simulink model "carModelMPC"  (R2020a)
settings: Solver=FixedStepAuto  StartTime=0.0  StopTime=time_length1  FixedStep=0.01  RelTol=1e-3
values from neighbouring files (symbols this model uses):
  c_s = 1450    [main_file.m]
  k_s = 30.01e+3    (= 30010)    [main_file.m]
  k_t = 3.4e5    (= 340000)    [main_file.m]
  m_s = 395.3    [main_file.m]
  m_u = 48.3    [main_file.m]
  P_dis = c2d(P,ts)    [main_file.m]
  ts = 0.01    [main_file.m]
undefined symbols (not defined in the file or in its folder): F_lim
settings Model: Creator=20183992  LastModifiedBy=Harold
settings DataIOCC: SaveFormat=Array  ReturnWorkspaceOutputs=off
settings DebuggingCC: ArithmeticOperatorsInVariantConditions=warning
settings SFSimCC: SimUseLocalCustomCode=off  CustomCodeUndefinedFunction=UseInterfaceOnly
settings RTWCC: RTWUseLocalCustomCode=off

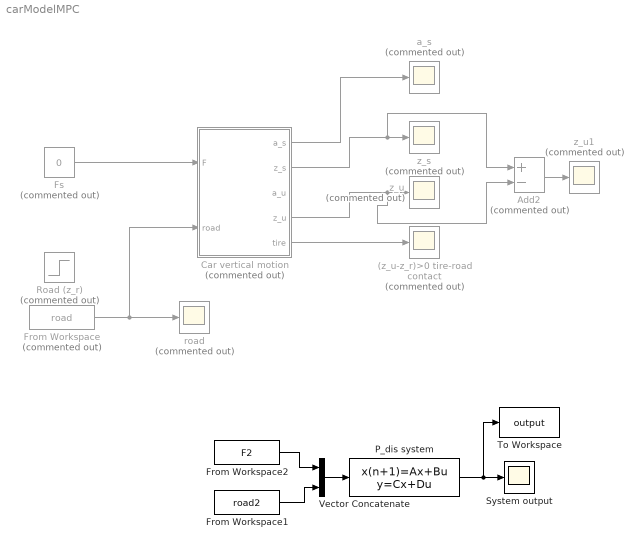
== system carModelMPC ==
  (z_u-z_r)>0 tire-road contact : Scope  Commented=on
  Add2 : Sum  Commented=on  Inputs=+-
  Car vertical motion : Subsystem  Commented=on
  From Workspace : FromWorkspace  Commented=on  VariableName=road  OutDataTypeStr=double  SampleTime=-1
  From Workspace1 : FromWorkspace  VariableName=road2  OutDataTypeStr=double  SampleTime=0.01
  From Workspace2 : FromWorkspace  VariableName=F2  OutDataTypeStr=double  SampleTime=0.01
  Fs : Constant  Commented=on  Value=0
  P_dis system : DiscreteStateSpace  A=P_dis.A  B=P_dis.B  C=P_dis.C  D=P_dis.D  SampleTime=ts
  Road (z_r) : Step  Commented=on  After=-0.1  SampleTime=0
  System output : Scope
  To Workspace : ToWorkspace  VariableName=output  SaveFormat=Timeseries  SampleTime=0.01
  Vector Concatenate : Concatenate  ConcatenateDimension=2
  a_s : Scope  Commented=on
  road : Scope  Commented=on
  z_s : Scope  Commented=on
  z_u : Scope  Commented=on
  z_u1 : Scope  Commented=on
  wires:
  Fs/1 -> Car vertical motion/1(F)
  Car vertical motion/5(tire) -> (z_u-z_r)>0 tire-road contact/1
  Car vertical motion/2(z_s) -> Add2/1, z_s/1
  Car vertical motion/4(z_u) -> Add2/2, z_u/1
  From Workspace/1 -> Car vertical motion/2(road), road/1
  Car vertical motion/1(a_s) -> a_s/1
  Add2/1 -> z_u1/1
  P_dis system/1 -> To Workspace/1, System output/1
  Vector Concatenate/1 -> P_dis system/1
  From Workspace1/1 -> Vector Concatenate/2
  From Workspace2/1 -> Vector Concatenate/1

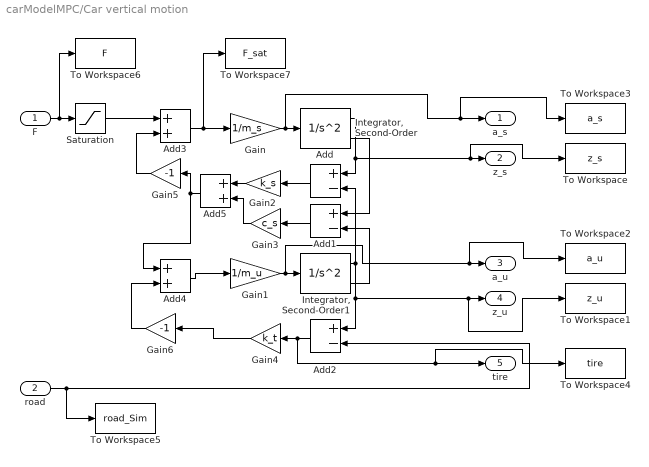
== system carModelMPC/Car vertical motion ==
  F : Inport
  road : Inport  Port=2
  Add : Sum  Inputs=+-
  Add1 : Sum  Inputs=+-
  Add2 : Sum  Inputs=+-
  Add3 : Sum
  Add4 : Sum
  Add5 : Sum
  Gain : Gain  Gain=1/m_s
  Gain1 : Gain  Gain=1/m_u
  Gain2 : Gain  Gain=k_s
  Gain3 : Gain  Gain=c_s
  Gain4 : Gain  Gain=k_t
  Gain5 : Gain  Gain=-1
  Gain6 : Gain  Gain=-1
  "Integrator, Second-Order" : SecondOrderIntegrator
  "Integrator, Second-Order1" : SecondOrderIntegrator
  Saturation : Saturate  UpperLimit=F_lim  LowerLimit=-F_lim
  To Workspace : ToWorkspace  VariableName=z_s  SaveFormat=Timeseries  SampleTime=-1
  To Workspace1 : ToWorkspace  VariableName=z_u  SaveFormat=Timeseries  SampleTime=-1
  To Workspace2 : ToWorkspace  VariableName=a_u  SaveFormat=Timeseries  SampleTime=-1
  To Workspace3 : ToWorkspace  VariableName=a_s  SaveFormat=Timeseries  SampleTime=-1
  To Workspace4 : ToWorkspace  VariableName=tire  SaveFormat=Timeseries  SampleTime=-1
  To Workspace5 : ToWorkspace  VariableName=road_Sim  SaveFormat=Timeseries  SampleTime=-1
  To Workspace6 : ToWorkspace  VariableName=F  SaveFormat=Timeseries  SampleTime=-1
  To Workspace7 : ToWorkspace  VariableName=F_sat  SaveFormat=Timeseries  SampleTime=-1
  a_s : Outport  VectorParamsAs1DForOutWhenUnconnected=off
  z_s : Outport  Port=2  VectorParamsAs1DForOutWhenUnconnected=off
  a_u : Outport  Port=3  VectorParamsAs1DForOutWhenUnconnected=off
  z_u : Outport  Port=4  VectorParamsAs1DForOutWhenUnconnected=off
  tire : Outport  Port=5  VectorParamsAs1DForOutWhenUnconnected=off
  wires:
  road/1 -> To Workspace5/1, Add2/2
  Gain/1 -> To Workspace3/1, a_s/1, "Integrator, Second-Order"/1
  "Integrator, Second-Order1"/2 -> Add1/2
  Add/1 -> Gain2/1
  "Integrator, Second-Order"/2 -> Add1/1
  Add2/1 -> To Workspace4/1, tire/1, Gain4/1
  Gain1/1 -> To Workspace2/1, a_u/1, "Integrator, Second-Order1"/1
  Gain3/1 -> Add5/2
  "Integrator, Second-Order"/1 -> To Workspace/1, z_s/1, Add/1
  Add4/1 -> Gain1/1
  Gain2/1 -> Add5/1
  Gain5/1 -> Add3/2
  Add3/1 -> To Workspace7/1, Gain/1
  Saturation/1 -> Add3/1
  Add1/1 -> Gain3/1
  Add5/1 -> Add4/1, Gain5/1
  Gain4/1 -> Gain6/1
  Gain6/1 -> Add4/2
  "Integrator, Second-Order1"/1 -> To Workspace1/1, z_u/1, Add2/1, Add/2
  F/1 -> To Workspace6/1, Saturation/1
